simulink model "Cuckoo Algoritm"  (R2019a)
settings: Solver=VariableStepAuto  StartTime=0.0  StopTime=1  MaxStep=1e-4  RelTol=1e-3
libraries: powerlib x17, re_lib x4, powerlib_meascontrol x1
settings Model: Creator=Mahesh Krishna  LastModifiedBy=ayubs
settings DataIOCC: ReturnWorkspaceOutputs=off
settings OptimizationCC: LifeSpan=inf
settings DebuggingCC: AlgebraicLoopMsg=none  ArithmeticOperatorsInVariantConditions=warning
settings SFSimCC: SimUseLocalCustomCode=off
settings RTWCC: RTWUseLocalCustomCode=off
settings CodeAppCC: StateflowObjectComments=on
settings SimscapeCC: SimscapeNormalizeSystem=off

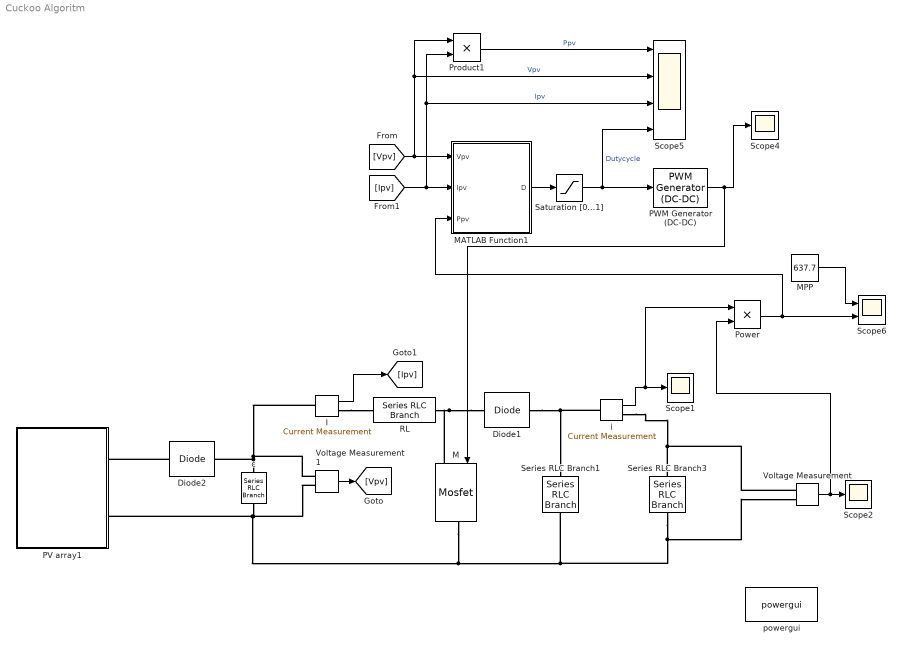
== system Cuckoo Algoritm ==
  Diode1 : powerlib/Power Electronics/Diode  Ron=1e-3  Lon=0  Vf=0  IC=0  UseSnubber=off  Rs=inf  Cs=inf  Measurements=off
      settings: SourceProductName=Simscape Electrical
  Diode2 : powerlib/Power Electronics/Diode  Ron=1e-3  Lon=0  Vf=0  IC=0  UseSnubber=off  Rs=inf  Cs=inf  Measurements=off
      settings: SourceProductName=Simscape Electrical
  I : powerlib/Measurements/Current Measurement  PhasorSimulation=off  OutputType=Magnitude  PSBequivalent=0
      settings: SourceProductName=Simscape Electrical
  M : powerlib/Power Electronics/Mosfet  Ron=1e-3  Lon=0  Rd=1e-3  Vfd=0  IC=0  Rs=inf  Cs=inf  Measurements=off
      settings: SourceProductName=Simscape Electrical
  MATLAB Function1 : MATLAB Function  TreatAsAtomicUnit=on
  MPP : Constant  Value=637.7
  PV array1 : Subsystem
  PWM Generator (DC-DC) : powerlib_meascontrol/Pulse & Signal Generators/PWM Generator (DC-DC)  Fsw=20e3  Ts=0
      settings: SourceProductName=Simscape Electrical
  Power : Product
  Product1 : Product
  RL : powerlib/Elements/Series RLC Branch  LConnTagsString=__new0  RConnTagsString=__new0  BranchType=L  Resistance=1e-3  Inductance=1.1478e-3  SetiL0=off  InitialCurrent=0  Capacitance=1e-6  Setx0=off  InitialVoltage=0  Measurements=None
      settings: SourceProductName=Simscape Electrical
  Saturation [0...1] : Saturate  UpperLimit=1  LowerLimit=0
  Scope1 : Scope
  Scope2 : Scope
  Scope4 : Scope
  Scope5 : Scope  NumInputPorts=4
  Scope6 : Scope  NumInputPorts=2
  Series RLC Branch1 : powerlib/Elements/Series RLC Branch  LConnTagsString=__new0  RConnTagsString=__new0  BranchType=C  Resistance=1e-4  Inductance=200e-6  SetiL0=off  InitialCurrent=0  Capacitance=0.4676e-3  Setx0=off  InitialVoltage=40  Measurements=None
      settings: SourceProductName=Simscape Electrical
  Series RLC Branch3 : powerlib/Elements/Series RLC Branch  LConnTagsString=__new0  RConnTagsString=__new0  BranchType=R  Resistance=100  Inductance=200e-6  SetiL0=off  InitialCurrent=0  Capacitance=1000e-6  Setx0=off  InitialVoltage=40  Measurements=None
      settings: SourceProductName=Simscape Electrical
  Voltage Measurement : powerlib/Measurements/Voltage Measurement  PhasorSimulation=off  OutputType=Magnitude  PSBequivalent=0
      settings: SourceProductName=Simscape Electrical
  Voltage Measurement1 : powerlib/Measurements/Voltage Measurement  PhasorSimulation=off  OutputType=Magnitude  PSBequivalent=0
      settings: SourceProductName=Simscape Electrical
  c : powerlib/Elements/Series RLC Branch  LConnTagsString=__new0  RConnTagsString=__new0  BranchType=C  Resistance=1e-3  Inductance=250e-6  SetiL0=off  InitialCurrent=0  Capacitance=10e-6  Setx0=off  InitialVoltage=0  Measurements=None
      settings: SourceProductName=Simscape Electrical
  i : powerlib/Measurements/Current Measurement  PhasorSimulation=off  OutputType=Magnitude  PSBequivalent=0
      settings: SourceProductName=Simscape Electrical
  powergui : powerlib/powergui  Priority=1  SimulationMode=Continuous  SampleTime=50e-6  frequency=60  Iterations=50  frequencyindice=0  Pbase=100e6  ErrMax=1e-4  UnitsV=kV  UnitsW=MW  buscounter=0  FunctionMessages=off  echomessages=off  EnableUseOfTLC=off  CurrentSourceSwitches=off  DisableSnubberDevices=off  DisableRonSwitches=off  DisableVfSwitches=off  DisplayEquations=off  AutomaticDiscreteSolvers=off  SolverType=Tustin/Backward Euler (TBE)  Interpol=off  ExternalGateDelay=off  methode=off  Ts=100  x0status=blocks  SPID=on  SwTol=0  HookPort=off  NonlinearTolerance=0  nMaxIteration=15  ContinueOnMaxIteration=off  RestoreLinks=warning  ResistiveCurrentMeasurement=off  Frange=[0:2:500]  Ylog=off  Xlog=on  ShowGrid=off  save=off  variable=ZData  structure=0  ZoomFFT=off  StartTime=0.0  cycles=1  DisplayStyle=1  fundamental=60  FreqAxis=off  MaxFrequency=1000  frequencyindicesteady=1  RmsSteady=1  display=off
      settings: SourceProductName=Simscape Electrical
  wires:
  I/1 -> [Ipv]
  [Ipv] -> MATLAB Function1/2(Ipv), Product1/2, Scope5/3  "Ipv"
  Voltage Measurement/1 -> Power/2, Scope2/1
  MATLAB Function1/1(D) -> Saturation [0...1]/1
  PWM Generator (DC-DC)/1 -> Scope4/1, M/1
  i/1 -> Power/1, Scope1/1
  Saturation [0...1]/1 -> Scope5/4, PWM Generator (DC-DC)/1  "Dutycycle"
  Voltage Measurement1/1 -> [Vpv]
  [Vpv] -> MATLAB Function1/1(Vpv), Product1/1, Scope5/2  "Vpv"
  MPP/1 -> Scope6/1
  Power/1 -> MATLAB Function1/3(Ppv), Scope6/2
  Product1/1 -> Scope5/1  "Ppv"
  connections:
  i/RConn1 -- Series RLC Branch3/LConn1 -- Voltage Measurement/LConn1
  Series RLC Branch1/RConn1 -- Series RLC Branch3/RConn1 -- Voltage Measurement/LConn2 -- Voltage Measurement1/LConn2 -- c/RConn1 -- PV array1/RConn2 -- M/RConn1
  Diode1/RConn1 -- Series RLC Branch1/LConn1 -- i/LConn1
  c/LConn1 -- Voltage Measurement1/LConn1 -- I/LConn1 -- Diode2/RConn1
  Diode1/LConn1 -- M/LConn1 -- RL/RConn1
  I/RConn1 -- RL/LConn1
  Diode2/LConn1 -- PV array1/RConn1

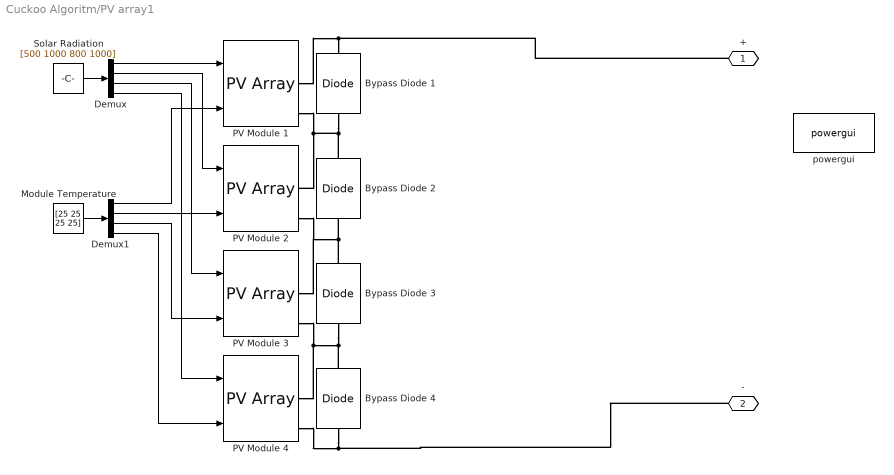
== system Cuckoo Algoritm/PV array1 ==
  Bypass Diode {1..4} (4 alike) : powerlib/Power Electronics/Diode  Ron=0.001  Lon=0  Vf=0.8  IC=0  UseSnubber=off  Rs=500  Cs=250e-9  Measurements=off
      settings: SourceProductName=Simscape Electrical
  Demux : Demux
  Demux1 : Demux
  Module Temperature : Constant  Value=[25 25 25 25]
  PV Module {1..4} (4 alike) : re_lib/Solar/PV Array  Npar=1  Nser=1  PlotType=array @ 1000 W/m2 & specified temperatures  S_vec="[ 1000  500  100 ]"  Temp_C_vec="[ 45 25  ]"  ModuleName=Tata Power Solar Systems TP250MBZ  PlotWhenSelected=off  Pm=249  Ncell=60  Voc=36.8  Isc=8.83  Vm=30  Im=8.3  beta_Voc_pc=-0.33  alpha_Isc_pc=0.063805  beta_Voc=-0.12144  alpha_Isc=0.005634  IL=8.8382  I0=1.0132e-10  nI=0.94812  Rsh=314.7646  Rs=0.2914  BAL=off  Tc=1e-6  Tfilter=5e-5
      settings: SourceProductName=Simscape Electrical
  Solar Radiation : Constant  Value=[500 1000 800 1000]
  powergui : powerlib/powergui  Priority=1  SimulationMode=Continuous  SampleTime=50e-6  frequency=60  Iterations=50  frequencyindice=0  Pbase=100e6  ErrMax=1e-4  UnitsV=kV  UnitsW=MW  buscounter=0  FunctionMessages=off  echomessages=off  EnableUseOfTLC=off  CurrentSourceSwitches=off  DisableSnubberDevices=off  DisableRonSwitches=off  DisableVfSwitches=off  DisplayEquations=off  AutomaticDiscreteSolvers=off  SolverType=Tustin/Backward Euler (TBE)  Interpol=off  ExternalGateDelay=off  methode=off  Ts=100  x0status=blocks  SPID=on  SwTol=0  HookPort=off  NonlinearTolerance=0  nMaxIteration=15  ContinueOnMaxIteration=off  RestoreLinks=warning  ResistiveCurrentMeasurement=off  Frange=[0:2:500]  Ylog=off  Xlog=on  ShowGrid=off  save=off  variable=ZData  structure=0  ZoomFFT=off  StartTime=0.0  cycles=1  DisplayStyle=1  fundamental=60  FreqAxis=off  MaxFrequency=1000  frequencyindicesteady=1  RmsSteady=1  display=off
      settings: SourceProductName=Simscape Electrical
  + : PMIOPort  Side=Right
  - : PMIOPort  Port=2  Side=Right
  wires:
  Solar Radiation/1 -> Demux/1
  Demux1/4 -> PV Module 4/2
  Demux/2 -> PV Module 2/1
  Module Temperature/1 -> Demux1/1
  Demux/3 -> PV Module 3/1
  Demux1/2 -> PV Module 2/2
  Demux/1 -> PV Module 1/1
  Demux1/1 -> PV Module 1/2
  Demux1/3 -> PV Module 3/2
  Demux/4 -> PV Module 4/1
  connections:
  Bypass Diode 3/RConn1 -- Bypass Diode 2/LConn1 -- PV Module 2/RConn2 -- PV Module 3/RConn1
  PV Module 3/RConn2 -- Bypass Diode 4/RConn1 -- Bypass Diode 3/LConn1 -- PV Module 4/RConn1
  Bypass Diode 2/RConn1 -- Bypass Diode 1/LConn1 -- PV Module 2/RConn1 -- PV Module 1/RConn2
  PV Module 1/RConn1 -- +/RConn1 -- Bypass Diode 1/RConn1
  Bypass Diode 4/LConn1 -- -/RConn1 -- PV Module 4/RConn2

== matlab function Cuckoo Algoritm/MATLAB Function1 ==
  settings: updateMethod=DISCRETE  sampleTime=1e-4
  data: Vpv input; D output; Ipv input; Ppv input
function D = Cuckoo(Vpv,Ipv,Ppv)
%#codegen
persistent u;
persistent dcurrent;
persistent p;
persistent dc;
persistent dbest;
persistent counter;
persistent iworst;
persistent discover;
if(isempty(discover))
    discover=0;
end
if(isempty(counter))
    counter=0;
end
if(isempty(dcurrent))
    dcurrent=0.5;
end
if(isempty(iworst))
    iworst=0;
end



if(isempty(dbest))
    dbest=0;
end
if(isempty(p))
    p=zeros(4,1);
end
if(isempty(u))
    u=0;
end
if(isempty(dc))
    dc=zeros(4,1);
    dc(1)=0;
    dc(2)=0.3;
    dc(3)=0.5;
    dc(4)=0.9;
end
if(counter>=1 && counter<150)
    D=dcurrent;
    counter=counter+1;
    return;
end
counter=0;

if(u>=1 && u<=4)
    p(u)=Vpv*Ipv;
    %p(u)=Ppv;
end
u=u+1;
if(u==7)
    u=1;
end
if(u==1)
    D=dc(u);
    dcurrent=D;
    counter=1;
    return;
elseif(u==2)
    D=dc(u);
    dcurrent=D;
    counter=1;
    return;
elseif(u==3)
    D=dc(u);
    dcurrent=D;
    counter=1;
    return;
elseif(u==4)
    D=dc(u);
    dcurrent=D;
    counter=1;
    return;
elseif(u==5 || u==6 )
    if(u==5)
        if(rand(1)>0.25)
            discover=1;
            [m,i]=max(p)
            dbest=dc(i);
            %determine the worst nest
            [m,iworst]=min(p);
            %build new nest
            %dc(iworst)=dbest;
            dc(iworst)=levyflight(dbest,dc(iworst));
            %dc(iworst)=withinlimits(dc(iworst));
            D=dc(iworst);
            dcurrent=D;
            counter=1;
            return;
        else
            u=u+1;
            [m,i]=max(p)
            dbest=dc(i);
            D=dbest;
            dcurrent=D;
            counter=1;
            dc(1)=levyflight(dbest,dc(1))
            % dc(1)=withinlimits(dc(1))
            dc(2)=levyflight(dbest,dc(2))
            %dc(2)=withinlimits(dc(2))
            dc(3)=levyflight(dbest,dc(3))
            % dc(3)=withinlimits(dc(3))
            dc(4)=levyflight(dbest,dc(4))
            % dc(4)=withinlimits(dc(4))
            return;
        end
        
    else
        %calculate new power of new nest
        p(iworst)=Vpv*Ipv;
        %p(iworst)=Ppv;
        %determine the best nest
        [m,i]=max(p);
        dbest=dc(i);
        D=dbest;
        dcurrent=D;
        counter=1;
        
        dc(1)=levyflight(dbest,dc(1))
        % dc(1)=withinlimits(dc(1))
        dc(2)=levyflight(dbest,dc(2))
        %dc(2)=withinlimits(dc(2))
        dc(3)=levyflight(dbest,dc(3))
        % dc(3)=withinlimits(dc(3))
        dc(4)=levyflight(dbest,dc(4))
        % dc(4)=withinlimits(dc(4))
        discover=0;
        return;
    end
    
else
    u
    y='hello'
    D=0.1
    
end


end
function dfinal=levyflight(dbest,d)
beta=3/2;
kcoeff=0.8;
sigmau=(gamma(1+beta)*sin(pi*beta/2)/(gamma((1+beta)/2)*beta*2^((beta-1)/2)))^(1/beta);
sigmav=1;
u=normrnd(0,(sigmau)^2);
v=normrnd(0,(sigmav)^2);
dup=d+(kcoeff*(abs(u)/((abs(v))^(1/beta)))*(dbest-d));


if(dup>1)
    dfinal=1;
elseif(dup<0)
    dfinal=0;
else
    dfinal=dup;
end
end
